simulink model "week2_1"  (R2020b)
settings: Solver=VariableStepAuto  StartTime=0.0  StopTime=inf  RelTol=1e-3
settings Model: Creator=Lenovo  LastModifiedBy=Lenovo

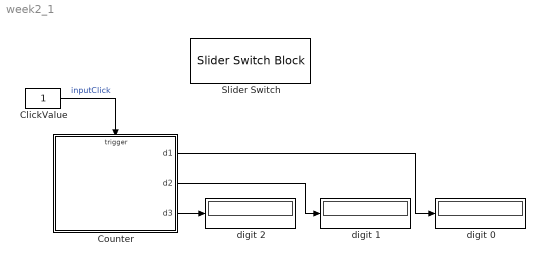
== system week2_1 ==
  ClickValue : Constant
  Counter : Stateflow chart  TreatAsAtomicUnit=on
  Slider Switch : SliderSwitchBlock  LabelPosition=Bottom
      settings: Values={{'Off', 'On'}, [0 1]}
  digit 0 : Display
  digit 1 : Display
  digit 2 : Display
  wires:
  Counter/2(d2) -> digit 1/1
  Counter/3(d3) -> digit 2/1
  Counter/1(d1) -> digit 0/1
  ClickValue/1 -> Counter/Trigger  "inputClick"

== stateflow chart week2_1/Counter ==
  settings: executeAtInitialization=1
  state digit1 [parallel]
    settings: executionOrder=1
    state zero
      en: d1 = 0;
    state one
      en: d1 = 1;
    digit1.zero -> digit1.one : inputClick
    (default) -> digit1.zero
    digit1.one -> digit1.zero : inputClick /{digit2.inc2;}
  state digit2 [parallel]
    settings: executionOrder=2
    state zero
      en: d2 = 0;
    state one
      en: d2 = 1;
    digit2.zero -> digit2.one : inc2
    (default) -> digit2.zero
    digit2.one -> digit2.zero : inc2 /{digit3.inc3;}
  state digit3 [parallel]
    settings: executionOrder=3
    state zero
      en: d3 = 0;
    state one
      en: d3 = 1;
    digit3.zero -> digit3.one : inc3
    (default) -> digit3.zero
    digit3.one -> digit3.zero : inc3
  data: d1 output size=1; d2 output size=1; d3 output size=1
  events: inc2 local EITHER_EDGE_EVENT; inc3 local EITHER_EDGE_EVENT; inputClick input EITHER_EDGE_EVENT
